simulink model "BLDC"  (R2020b)
settings: Solver=VariableStepAuto  StartTime=0.0  StopTime=2*pi  MaxStep=0.01  RelTol=1e-3
values from neighbouring files (symbols this model uses):
  J = 0.14    [BLDC_parameters.m]
  Lf = 0.1    [BLDC_parameters.m]
  Lff = 0.005    [BLDC_parameters.m]
  Md = 0    [BLDC_parameters.m]
  psi_f = 1    [BLDC_parameters.m]
  Rf = 10    [BLDC_parameters.m]
  Z = 1    [BLDC_parameters.m]
settings Model: Creator=Алексей  LastModifiedBy=Алексей

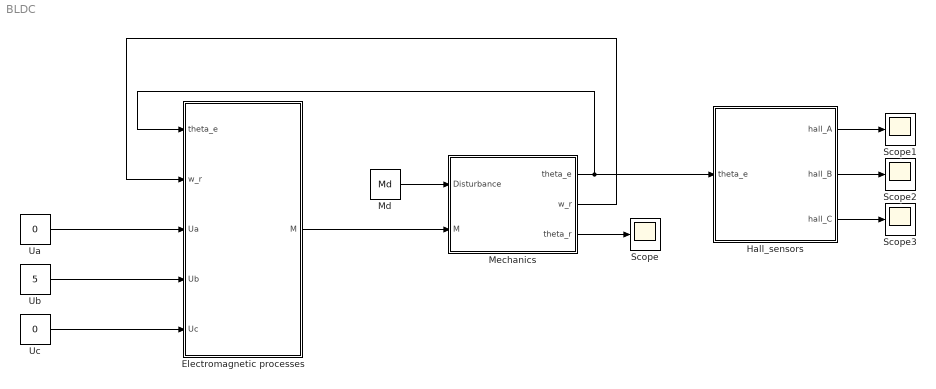
== system BLDC ==
  Electromagnetic processes : Subsystem
  Hall_sensors : MATLAB Function  TreatAsAtomicUnit=on
  Md : Constant  Value=Md
  Mechanics : Subsystem
  Scope{,1..3} (4 alike) : Scope
  Ua : Constant  Value=0
  Ub : Constant  Value=5
  Uc : Constant  Value=0
  wires:
  Mechanics/1(theta_e) -> Electromagnetic processes/1(theta_e), Hall_sensors/1(theta_e)
  Md/1 -> Mechanics/1(Disturbance)
  Mechanics/2(w_r) -> Electromagnetic processes/2(w_r)
  Ua/1 -> Electromagnetic processes/3(Ua)
  Ub/1 -> Electromagnetic processes/4(Ub)
  Uc/1 -> Electromagnetic processes/5(Uc)
  Electromagnetic processes/1(M) -> Mechanics/2(M)
  Mechanics/3(theta_r) -> Scope/1
  Hall_sensors/1(hall_A) -> Scope1/1
  Hall_sensors/2(hall_B) -> Scope2/1
  Hall_sensors/3(hall_C) -> Scope3/1

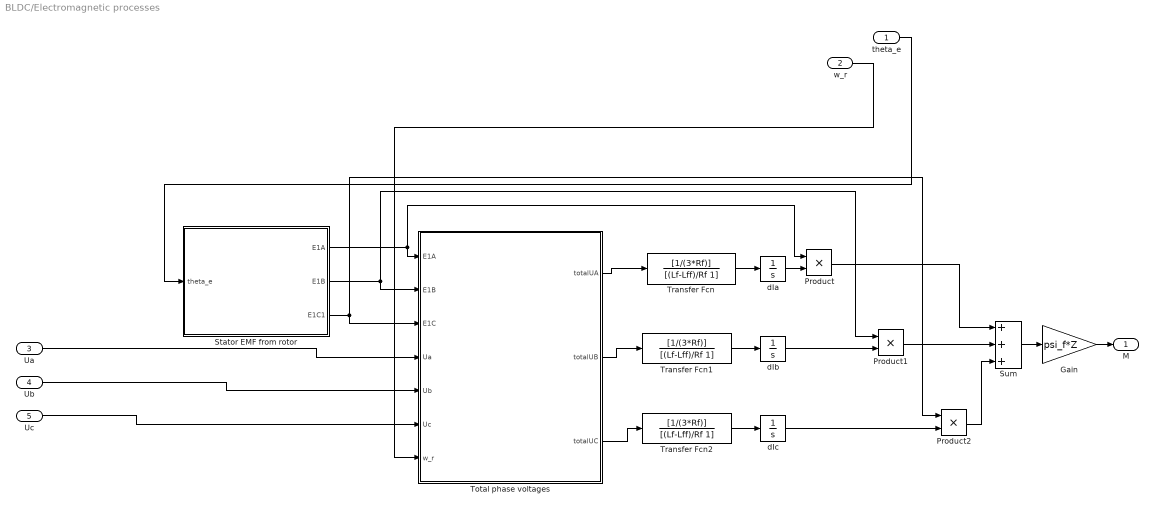
== system BLDC/Electromagnetic processes ==
  theta_e : Inport
  w_r : Inport  Port=2
  Ua : Inport  Port=3
  Ub : Inport  Port=4
  Uc : Inport  Port=5
  Gain : Gain  Gain=psi_f*Z
  Product : Product
  Product1 : Product
  Product2 : Product
  Stator EMF from rotor : Subsystem
  Sum : Sum  Inputs=+++
  Total phase voltages : MATLAB Function  TreatAsAtomicUnit=on
  Transfer Fcn : TransferFcn  Numerator=[1/(3*Rf)]  Denominator=[(Lf-Lff)/Rf 1]
  Transfer Fcn1 : TransferFcn  Numerator=[1/(3*Rf)]  Denominator=[(Lf-Lff)/Rf 1]
  Transfer Fcn2 : TransferFcn  Numerator=[1/(3*Rf)]  Denominator=[(Lf-Lff)/Rf 1]
  dIa : Integrator
  dIb : Integrator
  dIc : Integrator
  M : Outport
  wires:
  theta_e/1 -> Stator EMF from rotor/1(theta_e)
  Stator EMF from rotor/3(E1C1) -> Product2/1, Total phase voltages/3(E1C)
  Transfer Fcn2/1 -> dIc/1
  Total phase voltages/1(totalUA) -> Transfer Fcn/1
  Transfer Fcn/1 -> dIa/1
  Gain/1 -> M/1
  Stator EMF from rotor/1(E1A) -> Product/1, Total phase voltages/1(E1A)
  Product/1 -> Sum/1
  dIb/1 -> Product1/2
  Total phase voltages/3(totalUC) -> Transfer Fcn2/1
  Stator EMF from rotor/2(E1B) -> Product1/1, Total phase voltages/2(E1B)
  Uc/1 -> Total phase voltages/6(Uc)
  Product2/1 -> Sum/3
  Transfer Fcn1/1 -> dIb/1
  Total phase voltages/2(totalUB) -> Transfer Fcn1/1
  dIa/1 -> Product/2
  Product1/1 -> Sum/2
  dIc/1 -> Product2/2
  Sum/1 -> Gain/1
  Ua/1 -> Total phase voltages/4(Ua)
  w_r/1 -> Total phase voltages/7(w_r)
  Ub/1 -> Total phase voltages/5(Ub)

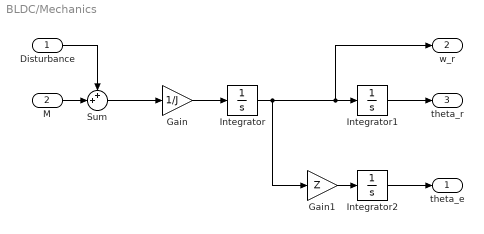
== system BLDC/Mechanics ==
  Disturbance : Inport
  M : Inport  Port=2
  Gain : Gain  Gain=1/J
  Gain1 : Gain  Gain=Z
  Integrator : Integrator
  Integrator1 : Integrator
  Integrator2 : Integrator
  Sum : Sum  Inputs=++|
  theta_e : Outport
  w_r : Outport  Port=2
  theta_r : Outport  Port=3
  wires:
  Gain/1 -> Integrator/1
  Integrator/1 -> Gain1/1, w_r/1, Integrator1/1
  Integrator1/1 -> theta_r/1
  M/1 -> Sum/2
  Sum/1 -> Gain/1
  Disturbance/1 -> Sum/1
  Gain1/1 -> Integrator2/1
  Integrator2/1 -> theta_e/1

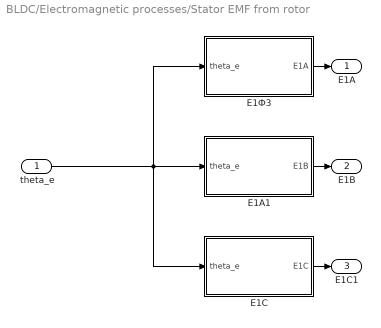
== system BLDC/Electromagnetic processes/Stator EMF from rotor ==
  theta_e : Inport
  E1A1 : MATLAB Function  TreatAsAtomicUnit=on
  E1C : MATLAB Function  TreatAsAtomicUnit=on
  E1Ф3 : MATLAB Function  TreatAsAtomicUnit=on
  E1A : Outport
  E1B : Outport  Port=2
  E1C1 : Outport  Port=3
  wires:
  theta_e/1 -> E1A1/1("theta_e "), E1C/1(theta_e), E1Ф3/1("theta_e ")
  E1A1/1(E1B) -> E1B/1
  E1C/1(E1C) -> E1C1/1
  E1Ф3/1(E1A) -> E1A/1

== matlab function BLDC/Electromagnetic processes/Stator EMF from rotor/E1A1 ==
  data: theta_e input; E1B output
function E1B = fcn(theta_e)
theta_e = mod(abs(theta_e), 2*pi);
if 0<=theta_e && theta_e<=pi/2
    E1B=1;
elseif pi/2<theta_e && theta_e<=5*pi/6
    E1B = -6/pi*(theta_e-4*pi/6);
elseif 5*pi/6<theta_e && theta_e<=9*pi/6
    E1B = -1;
elseif 9*pi/6<theta_e && theta_e<=11*pi/6
    E1B = 6/pi*(theta_e-10*pi/6);
else
    E1B = 1;
end

== matlab function BLDC/Electromagnetic processes/Stator EMF from rotor/E1Ф3 ==
  data: theta_e input; E1A output
function E1A = fcn(theta_e)
theta_e = mod(abs(theta_e), 2*pi);
if pi/6<=theta_e && theta_e<=5*pi/6
    E1A=-1;
elseif 7*pi/6<=theta_e && theta_e<=11*pi/6
    E1A=1;
elseif 0<=theta_e && theta_e<pi/6
    E1A=-6/pi*theta_e;
elseif 5*pi/6<theta_e && theta_e<7*pi/6
    E1A=6/pi*(theta_e - pi);
else
    E1A = -6/pi*(theta_e - 2*pi);
end

== matlab function BLDC/Electromagnetic processes/Stator EMF from rotor/E1C ==
  data: theta_e input; E1C output
function E1C = fcn(theta_e)
theta_e = mod(abs(theta_e), 2*pi);
if pi/2<=theta_e && theta_e<=7*pi/6
    E1C=1;
elseif pi/6<theta_e && theta_e<pi/2
    E1C=6/pi*(theta_e - 2*pi/6);
elseif 7*pi/6<theta_e && theta_e<9*pi/6
    E1C=-6/pi*(theta_e-8*pi/6);
else
    E1C = -1;
end

== matlab function BLDC/Hall_sensors ==
  data: theta_e input; hall_A output; hall_B output; hall_C output
function [hall_A, hall_B, hall_C] = fcn(theta_e)
theta_e = mod(abs(theta_e), 2*pi);
if pi/6<=theta_e && theta_e<=pi/2
    hall_A = 1;
    hall_B = 1;
    hall_C = 0;
elseif pi/2<theta_e && theta_e<=5*pi/6
    hall_A = 0;
    hall_B = 1;
    hall_C = 0;
elseif 5*pi/6<theta_e && theta_e<=7*pi/6
    hall_A = 0;
    hall_B = 1;
    hall_C = 1; 
elseif 7*pi/6<theta_e && theta_e<=3*pi/2
    hall_A = 0;
    hall_B = 0;
    hall_C = 1;
elseif 3*pi/2<theta_e && theta_e<=11*pi/6
    hall_A = 1;
    hall_B = 0;
    hall_C = 1;  
else
    hall_A = 1;
    hall_B = 0;
    hall_C = 0;
end

== matlab function BLDC/Electromagnetic processes/Total phase voltages ==
  data: E1A input; totalUA output; E1B input; E1C input; Ua input; Ub input; Uc input; w_r input; totalUB output; totalUC output; psi_f parameter; Z parameter
function [totalUA, totalUB, totalUC] = fcn(E1A, E1B, E1C, Ua, Ub, Uc, w_r, psi_f, Z)
totalUA=2*Ua-Ub-Uc+psi_f*Z*w_r*(E1B+E1C-2*E1A);
totalUB=2*Ub-Ua-Uc+psi_f*Z*w_r*(E1C+E1A-2*E1B);
totalUC=2*Uc-Ua-Ub+psi_f*Z*w_r*(E1A+E1B-2*E1C);
